simulink model "fig2_19b"  (Simulink 7.1)
settings: Solver=ode45  StartTime=0.0  StopTime=10.0  MaxStep=.05  MinStep=.01  RelTol=1e-3
settings Model: Creator=Office Depot  LastModifiedBy=Office Depot
settings SolverCC: InitialStep=.01

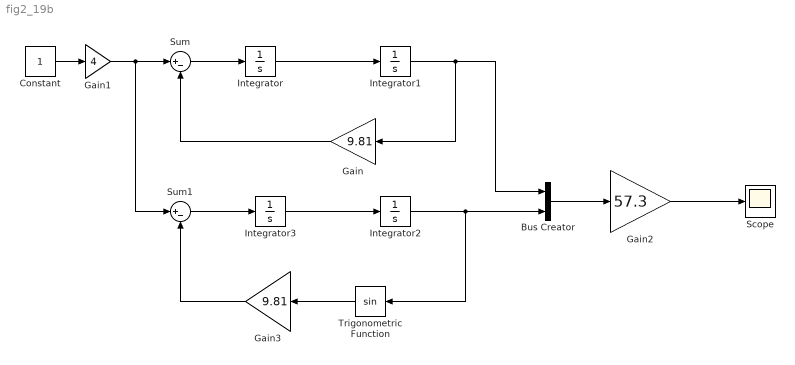
== system fig2_19b ==
  Bus Creator : BusCreator  Inputs=2
  Constant : Constant  OutDataType=sfix(16)  OutScaling=2^0
  Gain : Gain  Orientation=left  Gain=9.81  ParameterDataType=sfix(16)  ParameterScaling=2^0  OutDataType=sfix(16)  OutScaling=2^0
  Gain1 : Gain  Gain=4  ParameterDataType=sfix(16)  ParameterScaling=2^0  OutDataType=sfix(16)  OutScaling=2^0
  Gain2 : Gain  Gain=57.3  ParameterDataType=sfix(16)  ParameterScaling=2^0  OutDataType=sfix(16)  OutScaling=2^0
  Gain3 : Gain  Orientation=left  Gain=9.81  ParameterDataType=sfix(16)  ParameterScaling=2^0  OutDataType=sfix(16)  OutScaling=2^0
  Integrator{,1..3} (4 alike) : Integrator
  Scope : Scope
  Sum : Sum  Inputs=|+-  OutDataType=sfix(16)  OutScaling=2^0
  Sum1 : Sum  Inputs=|+-  OutDataType=sfix(16)  OutScaling=2^0
  Trigonometric Function : Trigonometry  Orientation=left
  wires:
  Integrator/1 -> Integrator1/1
  Integrator1/1 -> Gain/1, Bus Creator/1
  Sum/1 -> Integrator/1
  Gain/1 -> Sum/2
  Constant/1 -> Gain1/1
  Gain1/1 -> Sum/1, Sum1/1
  Integrator2/1 -> Bus Creator/2, Trigonometric Function/1
  Integrator3/1 -> Integrator2/1
  Sum1/1 -> Integrator3/1
  Bus Creator/1 -> Gain2/1
  Gain2/1 -> Scope/1
  Trigonometric Function/1 -> Gain3/1
  Gain3/1 -> Sum1/2
